simulink model "week2_ps4"  (R2020b)
settings: Solver=VariableStepAuto  StartTime=0.0  StopTime=0.2  RelTol=1e-3
values from neighbouring files (symbols this model uses):
  b = 3.5077E-6    [motordara.sldd]    (also in ps4.m = 3.5077e-06)
  J = 3.2284E-6    [motordara.sldd]    (also in ps4.m = 3.2284e-06)
  K = 0.0274    [motordara.sldd]    (also in ps4.m)
  L = 2.75E-6    [motordara.sldd]    (also in ps4.m = 2.75e-06)
  R = 4.0    [motordara.sldd]    (also in ps4.m = 4)
settings Model: DataDictionary=motordara.sldd  Creator=prana  LastModifiedBy=prana

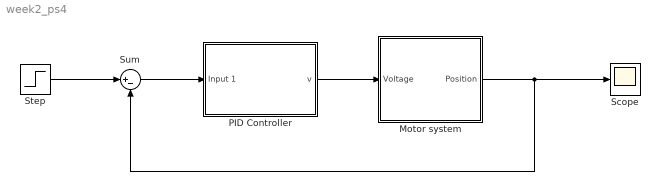
== system week2_ps4 ==
  Motor system : Subsystem
      mask Display: image('mmm.jfif'); % Use "Edit Image" on toolstrip to change.
  PID Controller : Subsystem  mask{Kp=21, Ki=500, Kd=0.15}
  Scope : Scope
  Step : Step  Time=0  After=500  SampleTime=0
  Sum : Sum  Inputs=|+-
  wires:
  Motor system/1(Position) -> Scope/1, Sum/2
  Step/1 -> Sum/1
  Sum/1 -> PID Controller/1(Input 1)
  PID Controller/1(v) -> Motor system/1(Voltage)

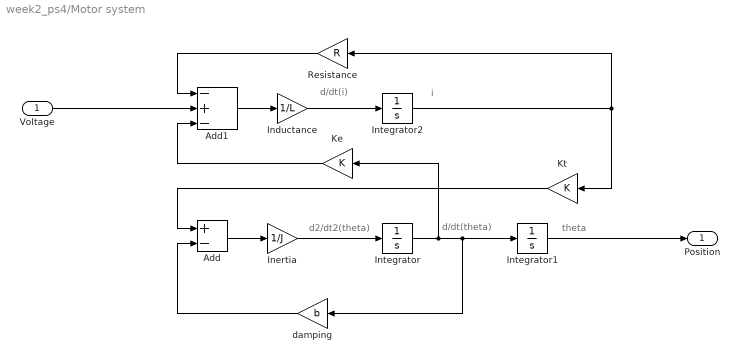
== system week2_ps4/Motor system ==
  note: theta
  note: d2/dt2(theta)
  note: d/dt(i)
  note: i
  note: d/dt(theta)
  Voltage : Inport
  Add : Sum  Inputs=+-
  Add1 : Sum  Inputs=-+-
  Inductance : Gain  Gain=1/L
  Inertia : Gain  Gain=1/J
  Integrator : Integrator
  Integrator1 : Integrator
  Integrator2 : Integrator
  Ke : Gain  Gain=K
  Kt : Gain  Gain=K
  Resistance : Gain  Gain=R
  damping : Gain  Gain=b
  Position : Outport
  wires:
  Ke/1 -> Add1/3
  Kt/1 -> Add/1
  Integrator/1 -> Ke/1, damping/1, Integrator1/1
  Add1/1 -> Inductance/1
  Inductance/1 -> Integrator2/1
  Integrator2/1 -> Resistance/1, Kt/1
  damping/1 -> Add/2
  Resistance/1 -> Add1/1
  Add/1 -> Inertia/1
  Inertia/1 -> Integrator/1
  Integrator1/1 -> Position/1
  Voltage/1 -> Add1/2

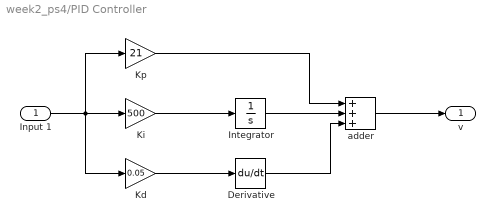
== system week2_ps4/PID Controller ==
  Input 1 : Inport
  Derivative : Derivative
  Integrator : Integrator
  Kd : Gain  Gain=0.05
  Ki : Gain  Gain=500
  Kp : Gain  Gain=21
  adder : Sum  Inputs=+++
  v : Outport
  wires:
  adder/1 -> v/1
  Ki/1 -> Integrator/1
  Input 1/1 -> Kd/1, Ki/1, Kp/1
  Kd/1 -> Derivative/1
  Derivative/1 -> adder/3
  Integrator/1 -> adder/2
  Kp/1 -> adder/1
